simulink model "PPS_Model"  (Simulink 8.2)
settings: Solver=FixedStepDiscrete  SolverMode=SingleTasking  StartTime=0.0  StopTime=inf  FixedStep=1/100  RelTol=1e-3
values from neighbouring files (symbols this model uses):
  dfreq = block.DialogPrm(1).Data    [msfcn_PPS_PlotSpeed.m]    (also in msfcn_PPS_radar_graph.m)
undefined symbols (not defined in the file or in its folder): gray, Rec, SDTV, strel
libraries: simulink x21, visiontextngfix x6, simulink_extras x3, visionsinks x2, visionconversions x2, visionstatistics x1, visionmorphops x1, visionanalysis x1
(part 1 of 2)
settings Model: Creator=Krzysztof  LastModifiedBy=raufk
settings DataIOCC: SaveOutput=off  SaveTime=off
settings OptimizationCC: InlineParams=on  OptimizeBlockIOStorage=off  BufferReuse=off  ExpressionFolding=off  LocalBlockOutputs=off  SimCompilerOptimization=On
settings DebuggingCC: ReadBeforeWriteMsg=DisableAll  WriteAfterWriteMsg=DisableAll  WriteAfterReadMsg=DisableAll  SolverPrmCheckMsg=none  MultiTaskDSMMsg=none  SigSpecEnsureSampleTimeMsg=none  ParameterPrecisionLossMsg=none  FrameProcessingCompatibilityMsg=error  UnknownTsInhSupMsg=none
settings ModelReferenceCC: ModelReferenceNumInstancesAllowed=Single
settings SFSimCC: SimParseCustomCode=off
settings GRTTargetCC: CodeReplacementLibrary=C89/C90 (ANSI)

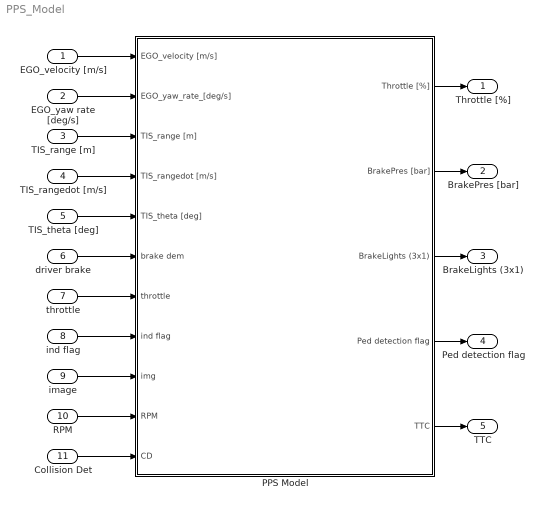
== system PPS_Model ==
  EGO_velocity [m/s] : Inport
  EGO_yaw rate [deg/s] : Inport  Port=2
  TIS_range [m] : Inport  Port=3
  TIS_rangedot [m/s] : Inport  Port=4
  TIS_theta [deg] : Inport  Port=5
  driver brake : Inport  Port=6
  throttle : Inport  Port=7
  ind flag : Inport  Port=8
  image : Inport  Port=9
  RPM : Inport  Port=10
  Collision Det : Inport  Port=11
  PPS Model : Subsystem  mask(PPS Model){MaxSpeed=70, MaxBrakePressure=150, BrakeDelay=100, LaneWidth=3.5, TISMaxRange=40, TISMaxTheta=60, TISfreq=25, TISdet=32, Camfreq=50, Mainfreq=100, DisplaySwitch=on, DisplayFreq=25, RadarSwitch=on, RadarFreq=25}
      mask prompts: MaxSpeed "Vehicle cut-off speed [km/h]"; MaxBrakePressure "Maximum value of braking pressure available [bar]"; BrakeDelay "Braking system delay [ms]"; LaneWidth "Lane width [m]"; TISMaxRange "TIS maximum range [m]"; TISMaxTheta "TIS maximum theta [deg]"; TISfreq "TIS frequency [Hz]"; TISdet "Max. number of Radar detected objects [-]"; Camfreq "Camera frequency [Hz]"; Mainfreq "Compilation sheet frequency [Hz]"; DisplaySwitch "Show EGO parameters visualization"; DisplayFreq "EGO parameters visualization frequency [Hz]"; RadarSwitch "Show radar visualization"; RadarFreq "Radar frequency [Hz]"
      mask help: PreScan Experiment and Pedestrian Protection System parameters
      mask Help: eval('openHelp(8130)')
      mask Callback DisplaySwitch:
      | en = get_param(gcb,'MaskEnables');
      | switch get_param(gcb, 'DisplaySwitch')
      |     case 'off'
      |         en{12} = 'off';
      |     case 'on'
      |         en{12} = 'on';
      | end
      | set_param(gcb,'MaskEnables',en);
      | clear en;
      mask Callback RadarSwitch:
      | en = get_param(gcb,'MaskEnables');
      | switch get_param(gcb, 'RadarSwitch')
      |     case 'off'
      |         en{14} = 'off';
      |     case 'on'
      |         en{14} = 'on';
      | end
      | set_param(gcb,'MaskEnables',en);
      | clear en;
  Throttle [%] : Outport
  BrakePres [bar] : Outport  Port=2
  BrakeLights (3x1) : Outport  Port=3
  Ped detection flag : Outport  Port=4
  TTC : Outport  Port=5
  wires:
  EGO_velocity [m/s]/1 -> PPS Model/1(EGO_velocity [m/s])
  EGO_yaw rate [deg/s]/1 -> PPS Model/2(EGO_yaw_rate_[deg/s])
  TIS_range [m]/1 -> PPS Model/3(TIS_range [m])
  TIS_rangedot [m/s]/1 -> PPS Model/4(TIS_rangedot [m/s])
  TIS_theta [deg]/1 -> PPS Model/5(TIS_theta [deg])
  throttle/1 -> PPS Model/7(throttle)
  ind flag/1 -> PPS Model/8(ind flag)
  image/1 -> PPS Model/9(img)
  PPS Model/1(Throttle [%]) -> Throttle [%]/1
  PPS Model/2(BrakePres [bar]) -> BrakePres [bar]/1
  PPS Model/3(BrakeLights (3x1)) -> BrakeLights (3x1)/1
  PPS Model/5(TTC) -> TTC/1
  driver brake/1 -> PPS Model/6(brake dem)
  RPM/1 -> PPS Model/10(RPM)
  Collision Det/1 -> PPS Model/11(CD)
  PPS Model/4(Ped detection flag) -> Ped detection flag/1

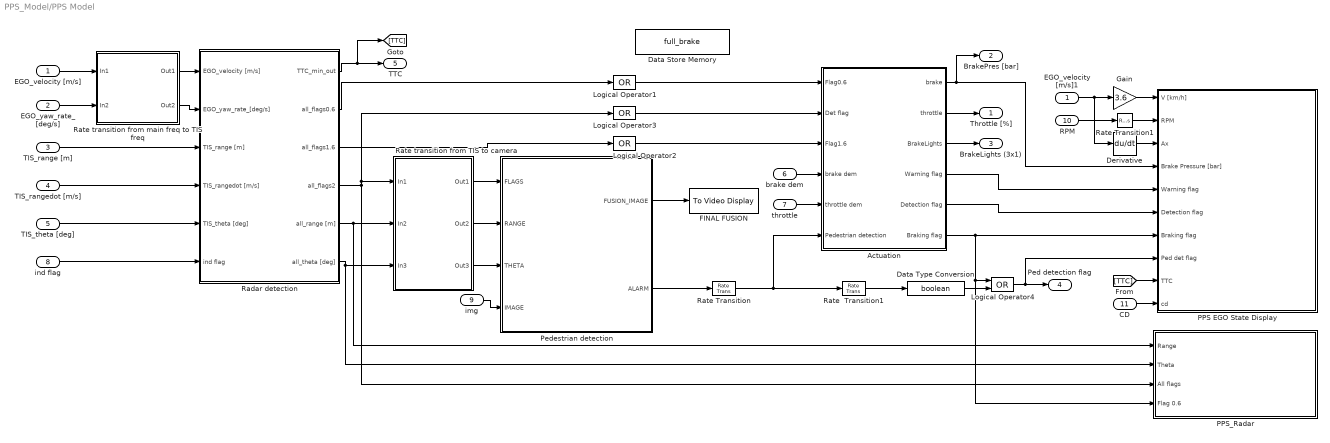
== system PPS_Model/PPS Model ==
  EGO_velocity [m/s] : Inport
  EGO_yaw_rate_[deg/s] : Inport  Port=2  SampleTime=1/Mainfreq
  TIS_range [m] : Inport  Port=3  PortDimensions=TISdet  SampleTime=1/TISfreq
  TIS_rangedot [m/s] : Inport  Port=4  PortDimensions=TISdet  SampleTime=1/TISfreq
  TIS_theta [deg] : Inport  Port=5  PortDimensions=TISdet  SampleTime=1/TISfreq
  brake dem : Inport  Port=6  SampleTime=[0,0]
  throttle : Inport  Port=7  SampleTime=[0,0]
  ind flag : Inport  Port=8  SampleTime=1/TISfreq
  img : Inport  Port=9  PortDimensions=[375 500]  SampleTime=1/Camfreq
  RPM : Inport  Port=10
  CD : Inport  Port=11
  Actuation : Subsystem
  Data Store Memory : DataStoreMemory  DataStoreName=full_brake  ReadBeforeWriteMsg=warning  WriteAfterWriteMsg=warning  WriteAfterReadMsg=warning
  Data Type Conversion : DataTypeConversion  OutDataTypeStr=boolean
  Derivative : Derivative
  EGO_velocity [m/s]1 : InportShadow
  FINAL FUSION : visionsinks/To Video Display  windowSizeMode=True size (1:1)  openAtMdlStart=on  fullScreen=off  videoWindowX=686  videoWindowY=98  saveWindowSize=off  videoWindowWidth=500  videoWindowHeight=375  inputColorFormat=RGB  inputType=Obsolete  imagePorts=One multidimensional signal  OutputDevice=On-screen video monitor  dataOrg=Column-major  isWindowOpen=off
  Gain : Gain  Gain=3.6
  Logical Operator1 : Logic  Operator=OR  Inputs=1  AllPortsSameDT=off  OutDataTypeStr=boolean
  Logical Operator2 : Logic  Operator=OR  Inputs=1  AllPortsSameDT=off  OutDataTypeStr=boolean
  Logical Operator3 : Logic  Operator=OR  Inputs=1  AllPortsSameDT=off  OutDataTypeStr=boolean
  Logical Operator4 : Logic  Operator=OR  AllPortsSameDT=off  OutDataTypeStr=boolean
  PPS EGO State Display : Subsystem  StopFcn=|
      | load('VRU_DisplaySwitch');
      | load('VRU_EGO_State_Coll');
      | load('VRU_EGO_State_BrakeVel');
      | load('VRU_EGO_State_Flag06');
      | s_VRU_DisplaySwitch = VRU_DisplaySwitch(2,end);
      | s_VRU_EGO_State_Coll = VRU_EGO_State_Coll(2,end);
      | s_VRU_EGO_State_BrakeVel = VRU_EGO_State_BrakeVel(2,end);
      | s_VRU_EGO_State_Flag06 = VRU_EGO_State_Flag06(2,end);
      | 
      | if(s_VRU_DisplaySwitch)
      |   CSpanel = findobj('Tag','cs_panel');
      |   CSvalue = findobj('Tag','cs_value');
      |   
      |   if(s_VRU_EGO_State_Coll)
      |      %Collision Occured
      |      set(CSpanel, 'BorderWidth',2, 'ForegroundColor',[0 120/255 0], 'HighlightColor',[0 120/255 0], 'ShadowColor', [0 120/255 0]);
      |      set(CSvalue, 'ForegroundColor',[0 120/255 0], 'String', strcat('Speed reduction', sprintf( ' %.1f ',s_VRU_EGO_State_BrakeVel-s_VRU_EGO_State_Coll), ' km/h'));
      |      set(CSpanel, 'Visible', 'On');
      |      set(CSvalue, 'Visible', 'On');
      |   else
      |     if(s_VRU_EGO_State_Flag06)
      |         % Collision almost occur
      |         set(CSpanel, 'BorderWidth',2, 'ForegroundColor','Green', 'HighlightColor','Green', 'ShadowColor', 'Green');
      |         set(CSvalue, 'ForegroundColor','Green', 'String', 'Collision avoided');
      |         set(CSpanel, 'Visible', 'On');
      |         set(CSvalue, 'Visible', 'On');
      |      else
      |         % No risk of collision
      |         set(CSpanel, 'Visible', 'Off');
      |         set(CSvalue, 'Visible', 'Off');
      |     end
      |   end
      | 
      |   clear CSpanel CSvalue
      | end
      | 
      | PPS_Speed_Profile
      | PPS_TTC_Profile
  PPS_Radar : Subsystem
  Pedestrian detection : Subsystem
  Radar detection : Subsystem
  Rate  Transition1 : RateTransition  Integrity=off  Deterministic=off  OutPortSampleTime=1/min(TISfreq,Camfreq)
  Rate Transition : RateTransition  Integrity=off  Deterministic=off  OutPortSampleTime=[0,0]
  Rate Transition1 : RateTransition  Integrity=off  Deterministic=off  OutPortSampleTime=1/Mainfreq
  Rate transition from TIS to camera : Subsystem
  Rate transition from main freq to TIS freq : Subsystem
  Throttle [%] : Outport
  BrakePres [bar] : Outport  Port=2
  BrakeLights (3x1) : Outport  Port=3
  Ped detection flag : Outport  Port=4  PortDimensions=1
  TTC : Outport  Port=5
  wires:
  TIS_range [m]/1 -> Radar detection/3(TIS_range [m])
  TIS_rangedot [m/s]/1 -> Radar detection/4(TIS_rangedot [m/s])
  TIS_theta [deg]/1 -> Radar detection/5(TIS_theta [deg])
  ind flag/1 -> Radar detection/6(ind flag)
  EGO_velocity [m/s]/1 -> Rate transition from main freq to TIS freq/1(In1)
  EGO_yaw_rate_[deg/s]/1 -> Rate transition from main freq to TIS freq/2(In2)
  Rate transition from main freq to TIS freq/1(Out1) -> Radar detection/1(EGO_velocity [m/s])
  Rate transition from main freq to TIS freq/2(Out2) -> Radar detection/2(EGO_yaw_rate_[deg/s])
  throttle/1 -> Actuation/5(throttle dem)
  brake dem/1 -> Actuation/4(brake dem)
  Radar detection/1(TTC_min_out) -> TTC/1, [TTC]
  Radar detection/2(all_flags0.6) -> Logical Operator1/1
  Rate Transition/1 -> Actuation/6(Pedestrian detection), Rate  Transition1/1
  Rate  Transition1/1 -> Data Type Conversion/1
  Radar detection/4(all_flags2) -> Rate transition from TIS to camera/1(In1), Logical Operator3/1, PPS_Radar/3(All flags)
  Radar detection/5(all_range [m]) -> Rate transition from TIS to camera/2(In2), PPS_Radar/1(Range)
  Radar detection/6(all_theta [deg]) -> PPS_Radar/2(Theta), Rate transition from TIS to camera/3(In3)
  Radar detection/3(all_flags1.6) -> Logical Operator2/1
  Actuation/1(brake) -> BrakePres [bar]/1, PPS EGO State Display/4(Brake Pressure [bar])
  Actuation/2(throttle) -> Throttle [%]/1
  Actuation/3(BrakeLights) -> BrakeLights (3x1)/1
  Actuation/6(Braking flag) -> PPS EGO State Display/7(Braking flag), Logical Operator4/1, PPS_Radar/4(Flag 0.6)
  img/1 -> Pedestrian detection/4(IMAGE)
  Pedestrian detection/1(FUSION_IMAGE) -> FINAL FUSION/1
  Rate transition from TIS to camera/1(Out1) -> Pedestrian detection/1(FLAGS)
  Rate transition from TIS to camera/2(Out2) -> Pedestrian detection/2(RANGE)
  Rate transition from TIS to camera/3(Out3) -> Pedestrian detection/3(THETA)
  Logical Operator1/1 -> Actuation/1(Flag0.6)
  Logical Operator2/1 -> Actuation/3(Flag1.6)
  Data Type Conversion/1 -> Logical Operator4/2
  Logical Operator4/1 -> PPS EGO State Display/8(Ped det flag), Ped detection flag/1
  Logical Operator3/1 -> Actuation/2(Det flag)
  EGO_velocity [m/s]1/1 -> Gain/1, Derivative/1
  Gain/1 -> PPS EGO State Display/1(V [km/h])
  RPM/1 -> Rate Transition1/1
  Derivative/1 -> PPS EGO State Display/3(Ax)
  CD/1 -> PPS EGO State Display/10(cd)
  [TTC] -> PPS EGO State Display/9(TTC)
  Actuation/4(Warning flag) -> PPS EGO State Display/5(Warning flag)
  Actuation/5(Detection flag) -> PPS EGO State Display/6(Detection flag)
  Rate Transition1/1 -> PPS EGO State Display/2(RPM)
  Pedestrian detection/2(ALARM) -> Rate Transition/1

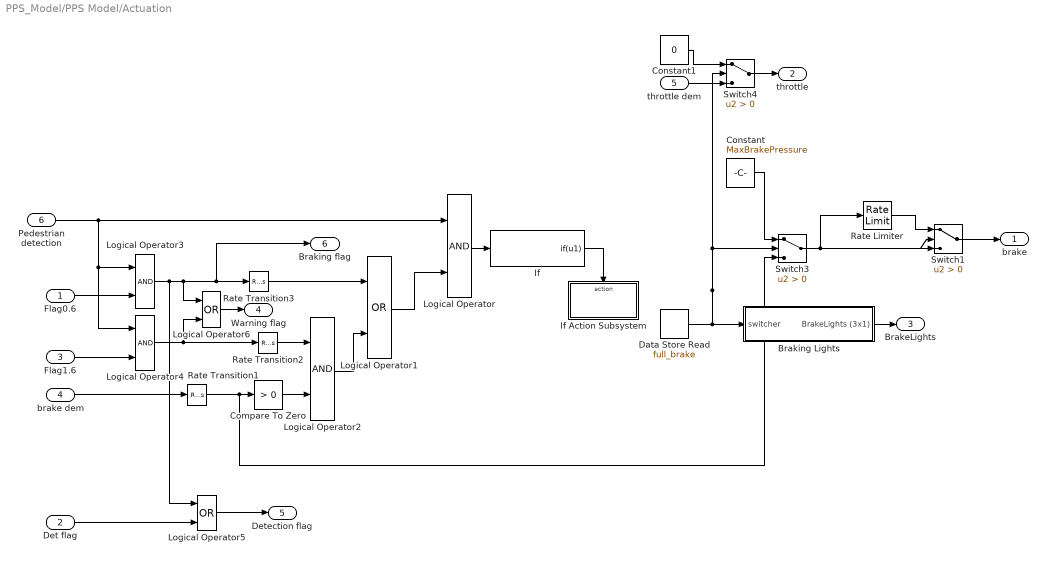
== system PPS_Model/PPS Model/Actuation ==
  Flag0.6 : Inport
  Det flag : Inport  Port=2
  Flag1.6 : Inport  Port=3
  brake dem : Inport  Port=4
  throttle dem : Inport  Port=5
  Pedestrian detection : Inport  Port=6
  Braking Lights : Subsystem
  Compare To Zero : simulink/Logic and Bit Operations/Compare To Zero  relop=>  OutDataTypeStr=uint8
  Constant : Constant  Value=MaxBrakePressure  SampleTime=[0,0]
  Constant1 : Constant  Value=0  SampleTime=[0,0]
  Data Store Read : DataStoreRead  DataStoreName=full_brake  SampleTime=1/Mainfreq
  If : If  IfExpression=u1  ShowElse=off
  If Action Subsystem : Subsystem  TreatAsAtomicUnit=on
  Logical Operator : Logic  AllPortsSameDT=off  OutDataTypeStr=boolean  SampleTime=[0,0]
  Logical Operator1 : Logic  Operator=OR  AllPortsSameDT=off  OutDataTypeStr=boolean  SampleTime=[0,0]
  Logical Operator2 : Logic  AllPortsSameDT=off  OutDataTypeStr=boolean  SampleTime=[0,0]
  Logical Operator3 : Logic  AllPortsSameDT=off  OutDataTypeStr=boolean  SampleTime=1/TISfreq
  Logical Operator4 : Logic  AllPortsSameDT=off  OutDataTypeStr=boolean  SampleTime=1/TISfreq
  Logical Operator5 : Logic  Operator=OR  AllPortsSameDT=off  OutDataTypeStr=boolean  SampleTime=1/TISfreq
  Logical Operator6 : Logic  Operator=OR  AllPortsSameDT=off  OutDataTypeStr=boolean  SampleTime=1/TISfreq
  Rate Limiter : RateLimiter  RisingSlewLimit=1000*0.9*MaxBrakePressure/BrakeDelay  FallingSlewLimit=-inf  SampleTimeMode=inherited
  Rate Transition1 : RateTransition  Integrity=off  OutPortSampleTime=[0,0]
  Rate Transition2 : RateTransition  Integrity=off  OutPortSampleTime=[0,0]
  Rate Transition3 : RateTransition  Integrity=off  OutPortSampleTime=[0,0]
  Switch1 : Switch  Criteria=u2 > Threshold  SampleTime=[0,0]
  Switch3 : Switch  Criteria=u2 > Threshold  SampleTime=[0,0]
  Switch4 : Switch  Criteria=u2 > Threshold  SampleTime=[0,0]
  brake : Outport  SampleTime=[0,0]
  throttle : Outport  Port=2  SampleTime=[0,0]
  BrakeLights : Outport  Port=3  SampleTime=1/Mainfreq
  Warning flag : Outport  Port=4
  Detection flag : Outport  Port=5
  Braking flag : Outport  Port=6
  wires:
  Pedestrian detection/1 -> Logical Operator3/1, Logical Operator4/1, Logical Operator/1
  Logical Operator1/1 -> Logical Operator/2
  Logical Operator2/1 -> Logical Operator1/2
  Compare To Zero/1 -> Logical Operator2/2
  Constant/1 -> Switch3/1
  Constant1/1 -> Switch4/1
  Switch4/1 -> throttle/1
  throttle dem/1 -> Switch4/3
  Braking Lights/1(BrakeLights (3x1)) -> BrakeLights/1
  brake dem/1 -> Rate Transition1/1
  Rate Transition1/1 -> Compare To Zero/1, Switch3/3
  Rate Transition2/1 -> Logical Operator2/1
  Rate Transition3/1 -> Logical Operator1/1
  Switch3/1 -> Switch1/3, Rate Limiter/1
  Rate Limiter/1 -> Switch1/1
  Switch1/1 -> brake/1
  Logical Operator3/1 -> Rate Transition3/1, Braking flag/1, Logical Operator6/1, Logical Operator5/1
  Logical Operator4/1 -> Rate Transition2/1, Logical Operator6/2
  Flag0.6/1 -> Logical Operator3/2
  Flag1.6/1 -> Logical Operator4/2
  Logical Operator6/1 -> Warning flag/1
  Det flag/1 -> Logical Operator5/2
  Logical Operator5/1 -> Detection flag/1
  Logical Operator/1 -> If/1
  Data Store Read/1 -> Braking Lights/1(switcher), Switch3/2, Switch1/2, Switch4/2
  If/1 -> If Action Subsystem/Action

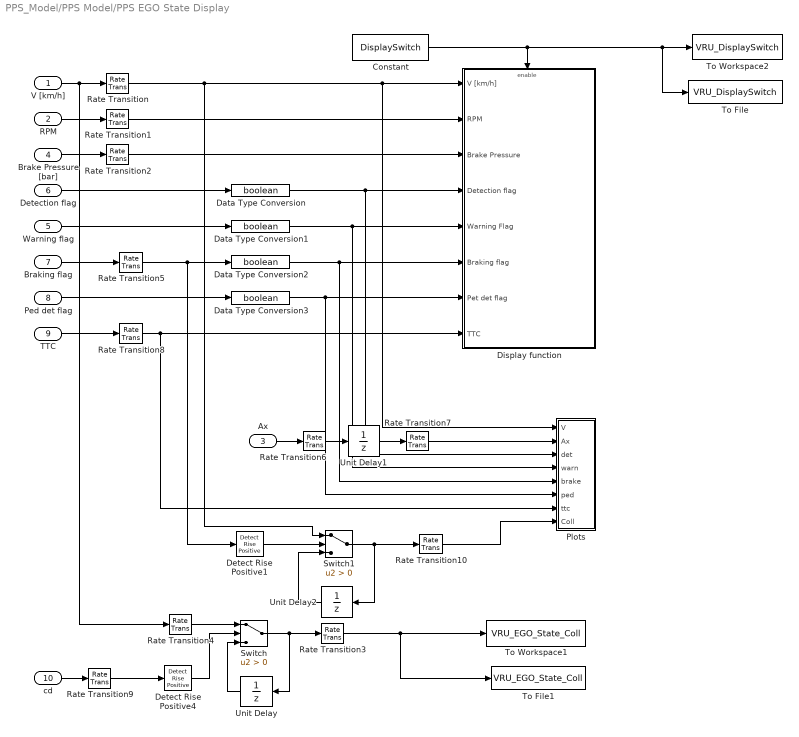
== system PPS_Model/PPS Model/PPS EGO State Display ==
  V [km/h] : Inport
  RPM : Inport  Port=2
  Ax : Inport  Port=3  SampleTime=[0,0]
  Brake Pressure [bar] : Inport  Port=4
  Warning flag : Inport  Port=5  OutDataTypeStr=boolean
  Detection flag : Inport  Port=6  OutDataTypeStr=boolean
  Braking flag : Inport  Port=7  OutDataTypeStr=boolean
  Ped det flag : Inport  Port=8  OutDataTypeStr=boolean
  TTC : Inport  Port=9
  cd : Inport  Port=10  OutDataTypeStr=boolean
  Constant : Constant  Value=DisplaySwitch
  Data Type Conversion{,1..3} (4 alike) : DataTypeConversion  OutDataTypeStr=boolean
  Detect Rise Positive1 : simulink/Logic and Bit Operations/Detect Rise Positive  vinit=0  InputProcessing=Inherited  OutDataTypeStr=uint8
  Detect Rise Positive4 : simulink/Logic and Bit Operations/Detect Rise Positive  vinit=0  InputProcessing=Inherited  OutDataTypeStr=uint8
  Display function : Subsystem
  Plots : Subsystem
      mask help:
      | The block calls functions:
      | * PPS_Speed_Profile
      | * PPS_TTC_Profile
      | to generate plots at the end of the simulation.
      | See stop callback of the block for more details.
  Rate Transition{,1..2,5,7..8} (6 alike) : RateTransition  Integrity=off  OutPortSampleTime=1/DisplayFreq
  Rate Transition10 : RateTransition  Integrity=off  OutPortSampleTime=[0,0]
  Rate Transition3 : RateTransition  Integrity=off  OutPortSampleTime=[0,0]
  Rate Transition4 : RateTransition  Integrity=off  OutPortSampleTime=1/Mainfreq
  Rate Transition6 : RateTransition  Integrity=off  OutPortSampleTimeOpt=Inherit  OutPortSampleTime=1/dfreq
  Rate Transition9 : RateTransition  Integrity=off  OutPortSampleTime=1/Mainfreq
  Switch : Switch  Criteria=u2 > Threshold  SampleTime=1/Mainfreq
  Switch1 : Switch  Criteria=u2 > Threshold  SampleTime=1/Mainfreq
  To File : ToFile  Filename=VRU_DisplaySwitch  MatrixName=VRU_DisplaySwitch  SampleTime=1/Mainfreq
  To File1 : ToFile  Filename=VRU_EGO_State_Coll  MatrixName=VRU_EGO_State_Coll  SampleTime=1/Mainfreq
  To Workspace1 : ToWorkspace  VariableName=VRU_EGO_State_Coll  SampleTime=1/Mainfreq
      settings: MaxDataPoints=1
  To Workspace2 : ToWorkspace  VariableName=VRU_DisplaySwitch  SampleTime=1/Mainfreq
      settings: MaxDataPoints=1
  Unit Delay : UnitDelay  SampleTime=1/Mainfreq
  Unit Delay1 : UnitDelay  SampleTime=-1
  Unit Delay2 : UnitDelay  SampleTime=1/Mainfreq
  wires:
  RPM/1 -> Rate Transition1/1
  Brake Pressure [bar]/1 -> Rate Transition2/1
  V [km/h]/1 -> Rate Transition/1, Rate Transition4/1
  Warning flag/1 -> Data Type Conversion1/1
  Ped det flag/1 -> Data Type Conversion3/1
  TTC/1 -> Rate Transition8/1
  Detection flag/1 -> Data Type Conversion/1
  Rate Transition/1 -> Display function/1(V [km/h]), Plots/1(V), Switch1/1
  Rate Transition1/1 -> Display function/2(RPM)
  Rate Transition3/1 -> To File1/1, To Workspace1/1
  cd/1 -> Rate Transition9/1
  Switch/1 -> Unit Delay/1, Rate Transition3/1
  Unit Delay/1 -> Switch/3
  Rate Transition4/1 -> Switch/1
  Detect Rise Positive4/1 -> Switch/2
  Braking flag/1 -> Rate Transition5/1
  Rate Transition5/1 -> Data Type Conversion2/1, Detect Rise Positive1/1
  Ax/1 -> Rate Transition6/1
  Unit Delay1/1 -> Rate Transition7/1
  Rate Transition6/1 -> Unit Delay1/1
  Rate Transition2/1 -> Display function/3(Brake Pressure)
  Rate Transition7/1 -> Plots/2(Ax)
  Rate Transition8/1 -> Plots/7(ttc), Display function/8(TTC)
  Rate Transition9/1 -> Detect Rise Positive4/1
  Data Type Conversion3/1 -> Plots/6(ped), Display function/7(Pet det flag)
  Data Type Conversion2/1 -> Display function/6(Braking flag), Plots/5(brake)
  Data Type Conversion1/1 -> Plots/4(warn), Display function/5(Warning Flag)
  Data Type Conversion/1 -> Plots/3(det), Display function/4(Detection flag)
  Constant/1 -> Display function/Enable, To File/1, To Workspace2/1
  Detect Rise Positive1/1 -> Switch1/2
  Switch1/1 -> Unit Delay2/1, Rate Transition10/1
  Unit Delay2/1 -> Switch1/3
  Rate Transition10/1 -> Plots/8(Coll)

== system PPS_Model/PPS Model/PPS_Radar ==
  Range : Inport
  Theta : Inport  Port=2
  All flags : Inport  Port=3  OutDataTypeStr=boolean
  Flag 0.6 : Inport  Port=4  OutDataTypeStr=boolean
  Constant : Constant  Value=RadarSwitch
  Radar : Subsystem
  Rate Transition{1..4} (4 alike) : RateTransition  Integrity=off  Deterministic=off  OutPortSampleTime=1/RadarFreq
  wires:
  Range/1 -> Rate Transition1/1
  Theta/1 -> Rate Transition2/1
  All flags/1 -> Rate Transition3/1
  Flag 0.6/1 -> Rate Transition4/1
  Rate Transition1/1 -> Radar/1(Range)
  Rate Transition2/1 -> Radar/2(Theta)
  Rate Transition3/1 -> Radar/3(All flags)
  Rate Transition4/1 -> Radar/4(Flag 0.6)
  Constant/1 -> Radar/Enable

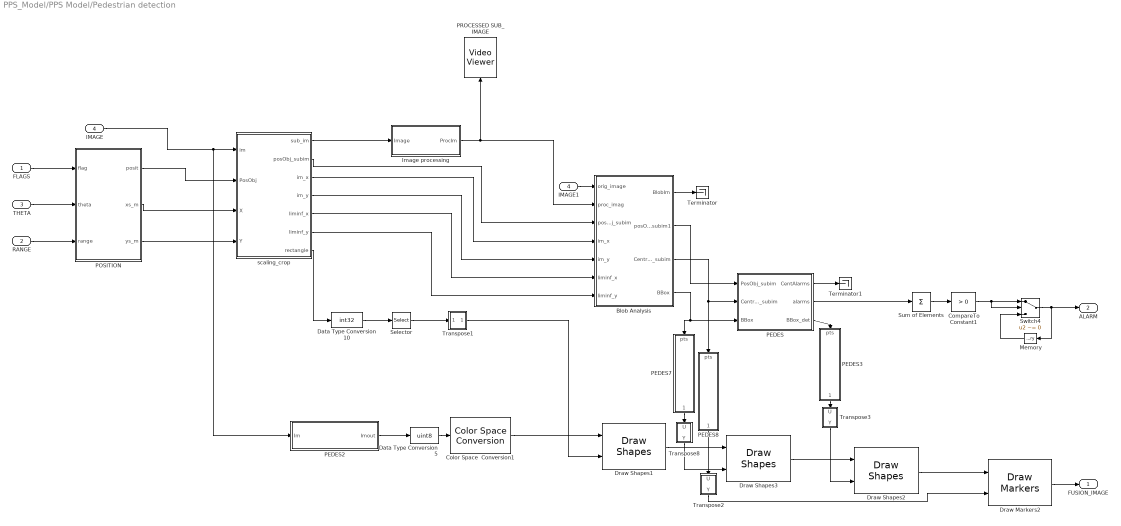
== system PPS_Model/PPS Model/Pedestrian detection ==
  FLAGS : Inport  OutDataTypeStr=boolean
  RANGE : Inport  Port=2  PortDimensions=TISdet
  THETA : Inport  Port=3
  IMAGE : Inport  Port=4  OutDataTypeStr=uint8  PortDimensions=[375 500]
  Blob Analysis : Subsystem
  Color Space  Conversion1 : visionconversions/Color Space  Conversion  conversion=Obsolete  conversionActive=Y'CbCr to R'G'B'  wp_str=D65  rec=Rec. 601 (SDTV)  sys=1125/60/2:1  imagePorts=One multidimensional signal
  CompareTo Constant1 : simulink/Logic and Bit Operations/Compare To Constant  relop=>  const=0  OutDataTypeStr=uint8
  Data Type Conversion10 : DataTypeConversion  OutDataTypeStr=int32
  Data Type Conversion5 : DataTypeConversion  OutDataTypeStr=uint8
  Draw Markers2 : visiontextngfix/Draw Markers  shape=X-mark  size=3  fill=on  fillClrSource=Specify via dialog  display=White  intensity=200  color=[200 255 100]  opacity=0.9  viewport=Entire image  antialiasing=on  inType=Obsolete  imagePorts=One multidimensional signal  prodOutputMode=Binary point scaling  prodOutputWordLength=32  prodOutputFracLength=14  memoryMode=Specify word length  memoryWordLength=16  memoryFracLength=14  roundingMode=Floor  overflowMode=off
  Draw Shapes1 : visiontextngfix/Draw Shapes  shape=Rectangles  fill=off  fillClrSource=Specify via dialog  display=White  intensity=200  color=[255 0 0]  opacity=0.5  viewport=Entire image  antialiasing=off  inType=Obsolete  imagePorts=One multidimensional signal  prodOutputMode=Binary point scaling  prodOutputWordLength=32  prodOutputFracLength=14  memoryMode=Specify word length  memoryWordLength=16  memoryFracLength=14  roundingMode=Floor  overflowMode=off
  Draw Shapes2 : visiontextngfix/Draw Shapes  shape=Rectangles  fill=on  fillClrSource=Specify via dialog  display=White  intensity=200  color=[255 0 0]  opacity=0.5  viewport=Entire image  antialiasing=off  inType=Obsolete  imagePorts=One multidimensional signal  prodOutputMode=Binary point scaling  prodOutputWordLength=32  prodOutputFracLength=14  memoryMode=Specify word length  memoryWordLength=16  memoryFracLength=14  roundingMode=Floor  overflowMode=off
  Draw Shapes3 : visiontextngfix/Draw Shapes  shape=Rectangles  fill=off  fillClrSource=Specify via dialog  display=User-specified value  intensity=200  color=[255 0 0]  opacity=0.5  viewport=Entire image  antialiasing=off  inType=Obsolete  imagePorts=One multidimensional signal  prodOutputMode=Binary point scaling  prodOutputWordLength=32  prodOutputFracLength=14  memoryMode=Specify word length  memoryWordLength=16  memoryFracLength=14  roundingMode=Floor  overflowMode=off
  IMAGE1 : InportShadow  Port=4  OutDataTypeStr=uint8  PortDimensions=[375 500]
  Image processing : Subsystem
  Memory : Memory
  PEDES : MATLAB Function  TreatAsAtomicUnit=on
      settings: PermitHierarchicalResolution=ParametersOnly
  PEDES2 : MATLAB Function  TreatAsAtomicUnit=on
      settings: PermitHierarchicalResolution=ParametersOnly
  PEDES3 : MATLAB Function  TreatAsAtomicUnit=on
      settings: PermitHierarchicalResolution=ParametersOnly
  PEDES7 : MATLAB Function  TreatAsAtomicUnit=on
      settings: PermitHierarchicalResolution=ParametersOnly
  PEDES8 : MATLAB Function  TreatAsAtomicUnit=on
      settings: PermitHierarchicalResolution=ParametersOnly
  POSITION : MATLAB Function  TreatAsAtomicUnit=on
      settings: PermitHierarchicalResolution=ParametersOnly
  PROCESSED SUB_IMAGE : visionsinks/Video Viewer  inputType=Obsolete7b  imagePorts=One multidimensional signal  useColorMap=off  colormapValue=gray(256)  specRange=off  minInputVal=0  maxInputVal=255  FigPos=[546 1020 501 324]  AxisZoom=on  trueSizedOnce=off  OpenAtMdlStart=on  DefaultConfigurationName=vipscopes.VideoViewerScopeCfg
  Selector : Selector  InputPortWidth=4  IndexOptions=Index vector (dialog)  Indices=[2, 1, 4, 3]  OutputSizes=1
  Sum of Elements : Sum  Inputs=+
  Switch4 : Switch  Criteria=u2 ~= 0
  Terminator : Terminator
  Terminator1 : Terminator
  Transpose1 : Subsystem
  Transpose2 : Subsystem
  Transpose3 : Subsystem
  Transpose8 : Subsystem
  scaling_crop : MATLAB Function  TreatAsAtomicUnit=on
      settings: PermitHierarchicalResolution=ParametersOnly
  FUSION_IMAGE : Outport
  ALARM : Outport  Port=2
  wires:
  THETA/1 -> POSITION/2(theta)
  FLAGS/1 -> POSITION/1(flag)
  RANGE/1 -> POSITION/3(range)
  Blob Analysis/3(Centroid_subim) -> PEDES/2(Centroid_subim), PEDES8/1(pts)
  PEDES/2(alarms) -> Sum of Elements/1
  Blob Analysis/4(BBox) -> PEDES/3(BBox), PEDES7/1(pts)
  Switch4/1 -> ALARM/1, Memory/1
  Memory/1 -> Switch4/3
  Sum of Elements/1 -> CompareTo Constant1/1
  CompareTo Constant1/1 -> Switch4/1, Switch4/2
  Blob Analysis/2(posObj_subim1) -> PEDES/1(PosObj_subim)
  scaling_crop/6(liminf_y) -> Blob Analysis/7(liminf_y)
  scaling_crop/7(rectangle) -> Data Type Conversion10/1
  PEDES2/1(Imout) -> Data Type Conversion5/1
  Data Type Conversion5/1 -> Color Space  Conversion1/1
  Color Space  Conversion1/1 -> Draw Shapes1/1
  Draw Shapes1/1 -> Draw Shapes3/1
  Draw Shapes3/1 -> Draw Shapes2/1
  Draw Shapes2/1 -> Draw Markers2/1
  POSITION/2(xs_m) -> scaling_crop/3(X)
  POSITION/3(ys_m) -> scaling_crop/4(Y)
  POSITION/1(posit) -> scaling_crop/2(PosObj)
  IMAGE/1 -> scaling_crop/1(im), PEDES2/1(Im)
  scaling_crop/1(sub_im) -> Image processing/1(Image)
  scaling_crop/2(posObj_subim) -> Blob Analysis/3(posObj_subim)
  scaling_crop/3(im_x) -> Blob Analysis/4(im_x)
  scaling_crop/4(im_y) -> Blob Analysis/5(im_y)
  scaling_crop/5(liminf_x) -> Blob Analysis/6(liminf_x)
  PEDES/3(BBox_det) -> PEDES3/1(pts)
  Draw Markers2/1 -> FUSION_IMAGE/1
  Image processing/1(ProcIm) -> Blob Analysis/2(proc_imag), PROCESSED SUB_IMAGE/1
  Transpose1/1(Y) -> Draw Shapes1/2
  Selector/1 -> Transpose1/1(U)
  Data Type Conversion10/1 -> Selector/1
  Transpose3/1(Y) -> Draw Shapes2/2
  Transpose2/1(Y) -> Draw Markers2/2
  Transpose8/1(Y) -> Draw Shapes3/2
  PEDES7/1(inpoints) -> Transpose8/1(U)
  PEDES8/1(inpoints) -> Transpose2/1(U)
  PEDES3/1(inpoints) -> Transpose3/1(U)
  Blob Analysis/1(BlobIm) -> Terminator/1
  PEDES/1(CentAlarms) -> Terminator1/1
  IMAGE1/1 -> Blob Analysis/1(orig_image)

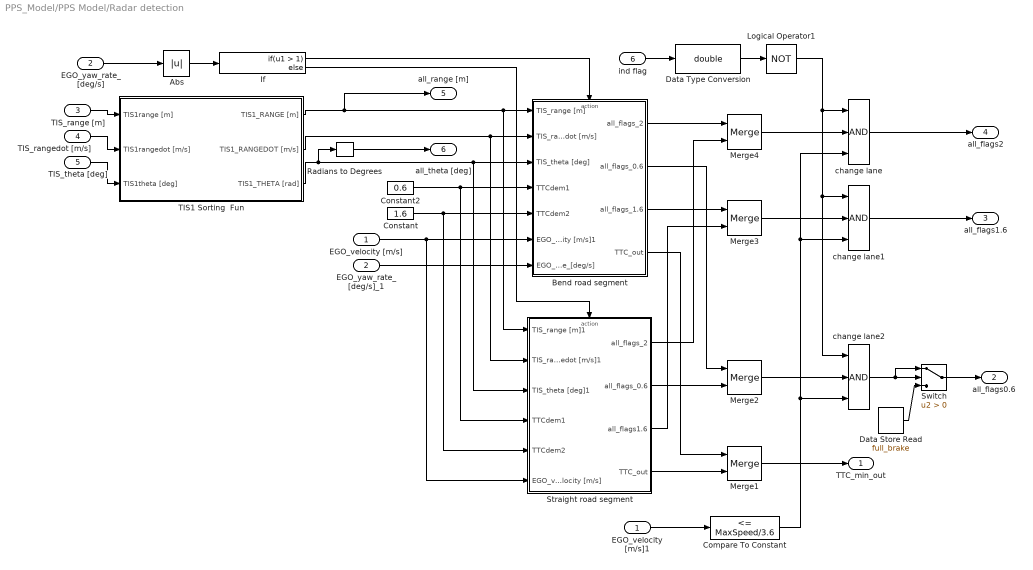
== system PPS_Model/PPS Model/Radar detection ==
  EGO_velocity [m/s] : Inport
  EGO_yaw_rate_[deg/s] : Inport  Port=2
  TIS_range [m] : Inport  Port=3  PortDimensions=TISdet
  TIS_rangedot [m/s] : Inport  Port=4  PortDimensions=TISdet
  TIS_theta [deg] : Inport  Port=5  PortDimensions=TISdet
  ind flag : Inport  Port=6
  Abs : Abs
  Bend road segment : Subsystem  TreatAsAtomicUnit=on
  Compare To Constant : simulink/Logic and Bit Operations/Compare To Constant  relop=<=  const=MaxSpeed/3.6  OutDataTypeStr=uint8
  Constant : Constant  Value=1.6
  Constant2 : Constant  Value=0.6
  Data Store Read : DataStoreRead  DataStoreName=full_brake  SampleTime=1/Mainfreq
  Data Type Conversion : DataTypeConversion  OutDataTypeStr=double
  EGO_velocity [m/s]1 : InportShadow
  EGO_yaw_rate_[deg/s]_1 : InportShadow  Port=2
  If : If  IfExpression=u1 > 1  SampleTime=1/TISfreq
  Logical Operator1 : Logic  Operator=NOT  AllPortsSameDT=off  OutDataTypeStr=boolean
  Merge{1..4} (4 alike) : Merge
  Radians to Degrees : simulink_extras/Transformations/Radians to Degrees
  Straight road segment : Subsystem  TreatAsAtomicUnit=on
  Switch : Switch  Criteria=u2 > Threshold
  TIS1 Sorting  Fun : Subsystem
  change lane : Logic  Inputs=3  AllPortsSameDT=off  OutDataTypeStr=boolean
  change lane1 : Logic  Inputs=3  AllPortsSameDT=off  OutDataTypeStr=boolean
  change lane2 : Logic  Inputs=3  AllPortsSameDT=off  OutDataTypeStr=boolean
  TTC_min_out : Outport
  all_flags0.6 : Outport  Port=2
  all_flags1.6 : Outport  Port=3
  all_flags2 : Outport  Port=4
  all_range [m] : Outport  Port=5
  all_theta [deg] : Outport  Port=6
  wires:
  TIS_range [m]/1 -> TIS1 Sorting  Fun/1(TIS1range [m])
  TIS_rangedot [m/s]/1 -> TIS1 Sorting  Fun/2(TIS1rangedot [m/s])
  TIS_theta [deg]/1 -> TIS1 Sorting  Fun/3(TIS1theta [deg])
  EGO_yaw_rate_[deg/s]/1 -> Abs/1
  If/1 -> Bend road segment/Action
  Abs/1 -> If/1
  TIS1 Sorting  Fun/1(TIS1_RANGE [m]) -> Bend road segment/1(TIS_range [m]), Straight road segment/1(TIS_range [m]1), all_range [m]/1
  TIS1 Sorting  Fun/2(TIS1_RANGEDOT [m/s]) -> Bend road segment/2(TIS_rangedot [m/s]), Straight road segment/2(TIS_rangedot [m/s]1)
  TIS1 Sorting  Fun/3(TIS1_THETA [rad]) -> Bend road segment/3(TIS_theta [deg]), Straight road segment/3(TIS_theta [deg]1), Radians to Degrees/1
  If/2 -> Straight road segment/Action
  Constant2/1 -> Bend road segment/4(TTCdem1), Straight road segment/4(TTCdem1)
  Constant/1 -> Bend road segment/5(TTCdem2), Straight road segment/5(TTCdem2)
  EGO_velocity [m/s]/1 -> Bend road segment/6(EGO_velocity [m/s]1), Straight road segment/6(EGO_velocity [m/s])
  EGO_yaw_rate_[deg/s]_1/1 -> Bend road segment/7(EGO_yaw_rate_[deg/s])
  ind flag/1 -> Data Type Conversion/1
  Bend road segment/2(all_flags_0.6) -> Merge2/1
  Straight road segment/2(all_flags_0.6) -> Merge2/2
  Straight road segment/3(all_flags1.6) -> Merge3/2
  Bend road segment/3(all_flags_1.6) -> Merge3/1
  Radians to Degrees/1 -> all_theta [deg]/1
  Data Type Conversion/1 -> Logical Operator1/1
  Straight road segment/4(TTC_out) -> Merge1/2
  Bend road segment/4(TTC_out) -> Merge1/1
  Merge1/1 -> TTC_min_out/1
  Bend road segment/1(all_flags_2) -> Merge4/1
  Straight road segment/1(all_flags_2) -> Merge4/2
  Merge4/1 -> change lane/2
  Logical Operator1/1 -> change lane/1, change lane2/1, change lane1/1
  Merge3/1 -> change lane1/2
  Merge2/1 -> change lane2/2
  change lane/1 -> all_flags2/1
  change lane2/1 -> Switch/2, Switch/1
  Switch/1 -> all_flags0.6/1
  EGO_velocity [m/s]1/1 -> Compare To Constant/1
  Compare To Constant/1 -> change lane2/3, change lane1/3, change lane/3
  change lane1/1 -> all_flags1.6/1
  Data Store Read/1 -> Switch/3

== system PPS_Model/PPS Model/Rate transition from TIS to camera ==
  In1 : Inport
  In2 : Inport  Port=2
  In3 : Inport  Port=3
  Rate Transition1 : RateTransition  Integrity=off  Deterministic=off  X0=zeros(TISdet,1)  OutPortSampleTime=1/Camfreq
  Rate Transition2 : RateTransition  Integrity=off  Deterministic=off  X0=zeros(TISdet,1)  OutPortSampleTime=1/Camfreq
  Rate Transition3 : RateTransition  Integrity=off  Deterministic=off  X0=zeros(TISdet,1)  OutPortSampleTime=1/Camfreq
  Out1 : Outport
  Out2 : Outport  Port=2
  Out3 : Outport  Port=3
  wires:
  In1/1 -> Rate Transition3/1
  In2/1 -> Rate Transition1/1
  In3/1 -> Rate Transition2/1
  Rate Transition3/1 -> Out1/1
  Rate Transition1/1 -> Out2/1
  Rate Transition2/1 -> Out3/1

== system PPS_Model/PPS Model/Rate transition from main freq to TIS freq ==
  In1 : Inport
  In2 : Inport  Port=2
  Rate Transition1 : RateTransition  Integrity=off  Deterministic=off  OutPortSampleTime=1/TISfreq
  Rate Transition2 : RateTransition  Integrity=off  Deterministic=off  OutPortSampleTime=1/TISfreq
  Out1 : Outport
  Out2 : Outport  Port=2
  wires:
  Rate Transition1/1 -> Out2/1
  In2/1 -> Rate Transition1/1
  In1/1 -> Rate Transition2/1
  Rate Transition2/1 -> Out1/1

== system PPS_Model/PPS Model/Actuation/Braking Lights ==
  note: === Braking lights block ===
      |
      |    - according to brake pressure, lights up braking lights of the actor,
      |    - the signal is a 3x1 vector:
      |      = first        value - left braking light,
      |      = second value - middle braking light,
      |      = third       value - right braking light.
  switcher : Inport
  Add : Sum
  Constant : Constant
  Constant1 : Constant  Value=0
  Mux : Mux  Inputs=3
  Pulse Generator : DiscretePulseGenerator  PulseType=Time based  Period=0.6  PulseWidth=50  PhaseDelay=0.3
  Rate Transition3 : RateTransition  Integrity=off  Deterministic=off  OutPortSampleTime=[0,0]
  Switch : Switch  Criteria=u2 > Threshold
  Switch1 : Switch  Criteria=u2 > Threshold
  Switch2 : Switch  Criteria=u2 > Threshold
  Unary Minus : UnaryMinus
  BrakeLights (3x1) : Outport
  wires:
  Mux/1 -> BrakeLights (3x1)/1
  switcher/1 -> Switch/2, Switch1/2, Switch2/2
  Constant/1 -> Switch/1, Add/2
  Switch/1 -> Switch1/3, Switch2/3, Mux/2
  Constant1/1 -> Switch/3
  Switch2/1 -> Mux/1
  Switch1/1 -> Mux/3
  Pulse Generator/1 -> Rate Transition3/1
  Add/1 -> Switch1/1
  Unary Minus/1 -> Add/1
  Rate Transition3/1 -> Unary Minus/1, Switch2/1

== system PPS_Model/PPS Model/Actuation/If Action Subsystem ==
  Action Port : ActionPort  ActionType=then
  Constant1 : Constant  SampleTime=[0,0]
  Data Store Write : DataStoreWrite  DataStoreName=full_brake
  wires:
  Constant1/1 -> Data Store Write/1

== system PPS_Model/PPS Model/PPS EGO State Display/Display function ==
  V [km/h] : Inport
  RPM : Inport  Port=2
  Brake Pressure : Inport  Port=3
  Detection flag : Inport  Port=4
  Warning Flag : Inport  Port=5
  Braking flag : Inport  Port=6
  Pet det flag : Inport  Port=7
  TTC : Inport  Port=8
  Enable : EnablePort
  Brake Pressure [bar]2 : Gain  Gain=100/MaxBrakePressure
  EGO Vehicle state display : M-S-Function  FunctionName=msfcn_PPS_PlotSpeed  Parameters=DisplayFreq DisplaySwitch
  Rounding Function2 : Rounding  Operator=round
  Rounding Function3 : Rounding  Operator=round
  wires:
  Brake Pressure [bar]2/1 -> Rounding Function3/1
  Rounding Function3/1 -> EGO Vehicle state display/3
  Rounding Function2/1 -> EGO Vehicle state display/2
  V [km/h]/1 -> EGO Vehicle state display/1
  Detection flag/1 -> EGO Vehicle state display/4
  Warning Flag/1 -> EGO Vehicle state display/5
  Braking flag/1 -> EGO Vehicle state display/6
  Pet det flag/1 -> EGO Vehicle state display/7
  TTC/1 -> EGO Vehicle state display/8
  RPM/1 -> Rounding Function2/1
  Brake Pressure/1 -> Brake Pressure [bar]2/1

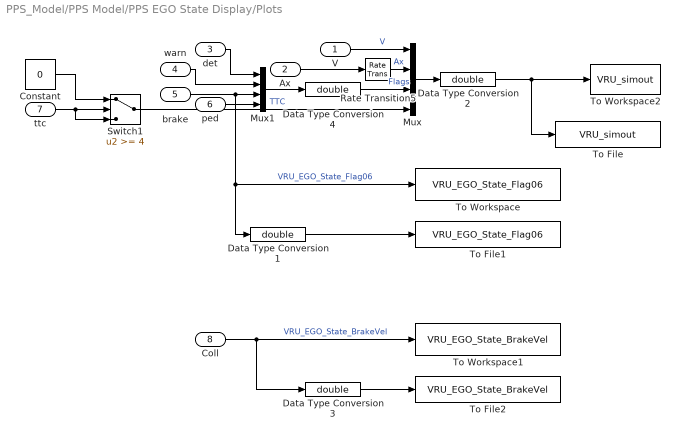
== system PPS_Model/PPS Model/PPS EGO State Display/Plots ==
  V : Inport
  Ax : Inport  Port=2  SampleTime=[0,0]
  det : Inport  Port=3
  warn : Inport  Port=4
  brake : Inport  Port=5
  ped : Inport  Port=6
  ttc : Inport  Port=7
  Coll : Inport  Port=8
  Constant : Constant  Value=0
  Data Type Conversion{1..4} (4 alike) : DataTypeConversion  OutDataTypeStr=double
  Mux : Mux
  Mux1 : Mux
  Rate Transition5 : RateTransition  Integrity=off  OutPortSampleTime=1/DisplayFreq
  Switch1 : Switch  Threshold=4
  To File : ToFile  Filename=VRU_simout  MatrixName=VRU_simout  SampleTime=1/Mainfreq
  To File1 : ToFile  Filename=VRU_EGO_State_Flag06  MatrixName=VRU_EGO_State_Flag06  SampleTime=1/Mainfreq
  To File2 : ToFile  Filename=VRU_EGO_State_BrakeVel  MatrixName=VRU_EGO_State_BrakeVel  SampleTime=1/Mainfreq
  To Workspace : ToWorkspace  VariableName=VRU_EGO_State_Flag06  SampleTime=-1
      settings: MaxDataPoints=1
  To Workspace1 : ToWorkspace  VariableName=VRU_EGO_State_BrakeVel  SampleTime=1/Mainfreq
      settings: MaxDataPoints=1
  To Workspace2 : ToWorkspace  VariableName=VRU_simout  SaveFormat=Structure With Time  SampleTime=0.04
  wires:
  Mux/1 -> Data Type Conversion2/1
  Mux1/1 -> Data Type Conversion4/1
  Data Type Conversion4/1 -> Mux/3  "Flags"
  Ax/1 -> Rate Transition5/1
  Rate Transition5/1 -> Mux/2  "Ax"
  Switch1/1 -> Mux/4  "TTC"
  Constant/1 -> Switch1/1
  V/1 -> Mux/1  "V"
  det/1 -> Mux1/1
  warn/1 -> Mux1/2
  brake/1 -> Mux1/3, Data Type Conversion1/1, To Workspace/1  "VRU_EGO_State_Flag06"
  ped/1 -> Mux1/4
  ttc/1 -> Switch1/2, Switch1/3
  Coll/1 -> Data Type Conversion3/1, To Workspace1/1  "VRU_EGO_State_BrakeVel"
  Data Type Conversion1/1 -> To File1/1
  Data Type Conversion2/1 -> To File/1, To Workspace2/1
  Data Type Conversion3/1 -> To File2/1

== system PPS_Model/PPS Model/PPS_Radar/Radar ==
  Range : Inport
  Theta : Inport  Port=2
  All flags : Inport  Port=3
  Flag 0.6 : Inport  Port=4
  Enable : EnablePort
  DISPLAY1 : M-S-Function  FunctionName=msfcn_PPS_radar_graph  Parameters=RadarFreq TISdet RadarSwitch TISMaxRange TISMaxTheta*pi/180
  Degrees to Radians : simulink_extras/Transformations/Degrees to Radians
  wires:
  Range/1 -> DISPLAY1/1
  Theta/1 -> Degrees to Radians/1
  All flags/1 -> DISPLAY1/3
  Flag 0.6/1 -> DISPLAY1/4
  Degrees to Radians/1 -> DISPLAY1/2

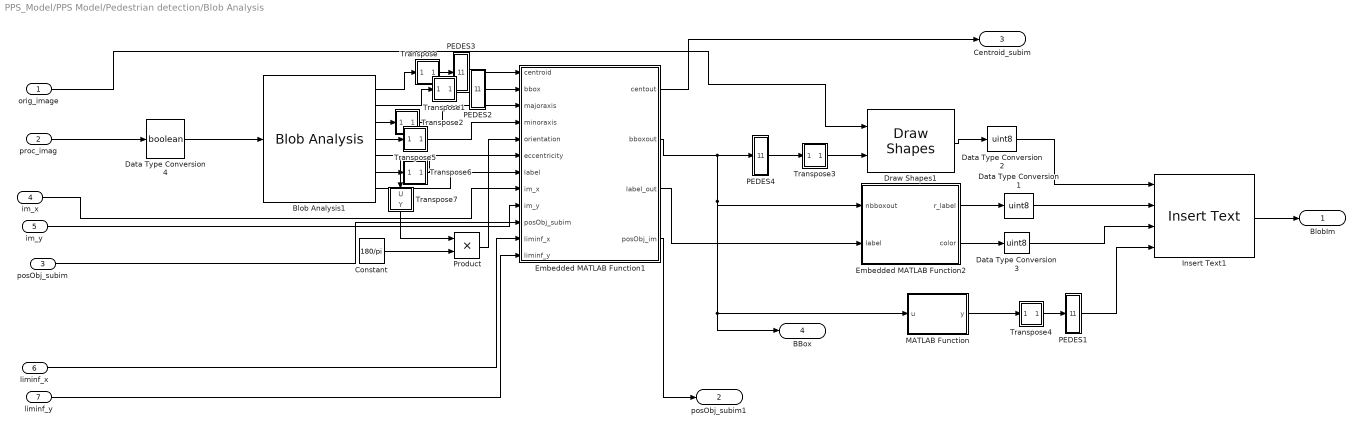
== system PPS_Model/PPS Model/Pedestrian detection/Blob Analysis ==
  orig_image : Inport
  proc_imag : Inport  Port=2
  posObj_subim : Inport  Port=3
  im_x : Inport  Port=4
  im_y : Inport  Port=5
  liminf_x : Inport  Port=6
  liminf_y : Inport  Port=7
  Blob Analysis1 : visionstatistics/Blob Analysis  Tag=vipblks_row_conv  area=off  centroid=on  bBox=on  majorAxis=on  minorAxis=on  angle=on  eccentricity=on  equivDiameterSq=off  extent=off  perimeter=off  maxBlobs=100  warnIfNumBlobsExceeded=on  isCount=off  useMinArea=on  minArea=50  useMaxArea=on  maxArea=150000  excludeBorderBlob=off  outDT=single  isOutVarDim=off  isFill=on  fillValues=-1  conn=4  isLabel=on  outputMode=Binary point scaling  outputWordLength=32  outputFracLength=16  firstCoeffMode=Binary point scaling  firstCoeffWordLength=16  firstCoeffFracLength=14  secondCoeffMode=Binary point scaling  secondCoeffWordLength=32  secondCoeffFracLength=16  accumMode=Binary point scaling  accumWordLength=32  accumFracLength=0  prodOutputMode=Binary point scaling  prodOutputWordLength=32  prodOutputFracLength=16  roundingMode=Floor  overflowMode=off
  Constant : Constant  Value=180/pi  VectorParams1D=off
  Data Type Conversion1 : DataTypeConversion  OutDataTypeStr=uint8
  Data Type Conversion2 : DataTypeConversion  OutDataTypeStr=uint8
  Data Type Conversion3 : DataTypeConversion  OutDataTypeStr=uint8
  Data Type Conversion4 : DataTypeConversion  OutDataTypeStr=boolean
  Draw Shapes1 : visiontextngfix/Draw Shapes  shape=Rectangles  fill=off  fillClrSource=Specify via dialog  display=White  intensity=200  color=[200 255 100]  opacity=0.6  viewport=Entire image  antialiasing=off  inType=Obsolete  imagePorts=One multidimensional signal  prodOutputMode=Binary point scaling  prodOutputWordLength=32  prodOutputFracLength=14  memoryMode=Specify word length  memoryWordLength=16  memoryFracLength=15  roundingMode=Floor  overflowMode=off
  Embedded MATLAB Function1 : MATLAB Function  TreatAsAtomicUnit=on
      settings: PermitHierarchicalResolution=ParametersOnly
  Embedded MATLAB Function2 : MATLAB Function  TreatAsAtomicUnit=on
      settings: PermitHierarchicalResolution=ParametersOnly
  Insert Text1 : visiontextngfix/Insert Text  inputType=Obsolete  theText='%02d'  getTextLocFrom=Input port  textLoc=[1 1]  getTextColorFrom=Input port  textColor=[0 0 0]  getTextIntensityFrom=Specify via dialog  textIntensity=0  getTextOpacityFrom=Specify via dialog  textOpacity=1.0  dummyVar2=0  dummyVar3=0  dummyVar4=0  imagePorts=One multidimensional signal  isInputTransposed=off  fontFace=LucidaSansRegular  dummyVar1=0  blockFontSize=12  antiAliased=on
  MATLAB Function : MATLAB Function  TreatAsAtomicUnit=on
      settings: PermitHierarchicalResolution=ParametersOnly
  PEDES1 : MATLAB Function  TreatAsAtomicUnit=on
      settings: PermitHierarchicalResolution=ParametersOnly
  PEDES2 : MATLAB Function  TreatAsAtomicUnit=on
      settings: PermitHierarchicalResolution=ParametersOnly
  PEDES3 : MATLAB Function  TreatAsAtomicUnit=on
      settings: PermitHierarchicalResolution=ParametersOnly
  PEDES4 : MATLAB Function  TreatAsAtomicUnit=on
      settings: PermitHierarchicalResolution=ParametersOnly
  Product : Product  RndMeth=Zero
  Transpose : Subsystem
  Transpose1 : Subsystem
  Transpose2 : Subsystem
  Transpose3 : Subsystem
  Transpose4 : Subsystem
  Transpose5 : Subsystem
  Transpose6 : Subsystem
  Transpose7 : Subsystem
  BlobIm : Outport
  posObj_subim1 : Outport  Port=2
  Centroid_subim : Outport  Port=3
  BBox : Outport  Port=4
  wires:
  Blob Analysis1/4 -> Transpose5/1(U)
  Constant/1 -> Product/2
  Embedded MATLAB Function2/1(r_label) -> Data Type Conversion1/1
  Embedded MATLAB Function2/2(color) -> Data Type Conversion3/1
  Draw Shapes1/1 -> Data Type Conversion2/1
  Data Type Conversion1/1 -> Insert Text1/2
  Data Type Conversion2/1 -> Insert Text1/1
  Data Type Conversion3/1 -> Insert Text1/3
  Blob Analysis1/1 -> Transpose/1(U)
  Blob Analysis1/2 -> Transpose1/1(U)
  Blob Analysis1/3 -> Transpose2/1(U)
  Blob Analysis1/5 -> Transpose7/1(U)
  Product/1 -> Embedded MATLAB Function1/5(orientation)
  Blob Analysis1/7 -> Embedded MATLAB Function1/7(label)
  Embedded MATLAB Function1/3(label_out) -> Embedded MATLAB Function2/2(label)
  Embedded MATLAB Function1/2(bboxout) -> Embedded MATLAB Function2/1(nbboxout), BBox/1, MATLAB Function/1(u), PEDES4/1(pts)
  Embedded MATLAB Function1/1(centout) -> Centroid_subim/1
  Insert Text1/1 -> BlobIm/1
  proc_imag/1 -> Data Type Conversion4/1
  im_x/1 -> Embedded MATLAB Function1/8(im_x)
  orig_image/1 -> Draw Shapes1/1
  im_y/1 -> Embedded MATLAB Function1/9(im_y)
  liminf_x/1 -> Embedded MATLAB Function1/11(liminf_x)
  liminf_y/1 -> Embedded MATLAB Function1/12(liminf_y)
  posObj_subim/1 -> Embedded MATLAB Function1/10(posObj_subim)
  Embedded MATLAB Function1/4(posObj_im) -> posObj_subim1/1
  Data Type Conversion4/1 -> Blob Analysis1/1
  Blob Analysis1/6 -> Transpose6/1(U)
  PEDES1/1(inpoints) -> Insert Text1/4
  Transpose/1(Y) -> PEDES3/1(pts)
  Transpose1/1(Y) -> PEDES2/1(pts)
  Transpose3/1(Y) -> Draw Shapes1/2
  PEDES2/1(inpoints) -> Embedded MATLAB Function1/2(bbox)
  PEDES3/1(inpoints) -> Embedded MATLAB Function1/1(centroid)
  Transpose4/1(Y) -> PEDES1/1(pts)
  PEDES4/1(inpoints) -> Transpose3/1(U)
  Transpose7/1(Y) -> Product/1
  Transpose6/1(Y) -> Embedded MATLAB Function1/6(eccentricity)
  Transpose5/1(Y) -> Embedded MATLAB Function1/4(minoraxis)
  Transpose2/1(Y) -> Embedded MATLAB Function1/3(majoraxis)
  MATLAB Function/1(y) -> Transpose4/1(U)

== system PPS_Model/PPS Model/Pedestrian detection/Image processing ==
  Image : Inport
  Closing : visionmorphops/Closing  nhoodsrc=Specify via dialog  strel=strel('disk', 4)
  Edge Detection : visionanalysis/Edge Detection  method=Canny  outputType=Binary image  userDefinedThreshold=off  thresholdSource=Specify via dialog  threshold=1  thresholdTuning=3  edgeThinning=off  threshold_canny=[0.25 0.60]  autoPercent=93  sigma=1  prodOutputMode=Binary point scaling  prodOutputWordLength=32  prodOutputFracLength=8  roundingMode=Floor  overflowMode=off
  Embedded MATLAB Function : MATLAB Function  TreatAsAtomicUnit=on
      settings: PermitHierarchicalResolution=ParametersOnly
  Image Data Type Conversion1 : visionconversions/Image Data Type Conversion  outDT=single  isSigned=on  wordLen=16  numFracBits=0
  ProcIm : Outport
  wires:
  Closing/1 -> Embedded MATLAB Function/1(image)
  Embedded MATLAB Function/1(im) -> ProcIm/1
  Image/1 -> Image Data Type Conversion1/1
  Edge Detection/1 -> Closing/1
  Image Data Type Conversion1/1 -> Edge Detection/1

== system PPS_Model/PPS Model/Pedestrian detection/Transpose1 ==
  U : Inport
  Data Type Conversion : DataTypeConversion
  Data Type Conversion1 : DataTypeConversion
  Interpreted MATLAB Function : MATLABFcn  MATLABFcn=transpose  Output1D=off
  Y : Outport
  wires:
  Data Type Conversion1/1 -> Y/1
  Interpreted MATLAB Function/1 -> Data Type Conversion1/1
  Data Type Conversion/1 -> Interpreted MATLAB Function/1
  U/1 -> Data Type Conversion/1

== system PPS_Model/PPS Model/Pedestrian detection/Transpose2 ==
  U : Inport
  Data Type Conversion : DataTypeConversion
  Data Type Conversion1 : DataTypeConversion
  Interpreted MATLAB Function : MATLABFcn  MATLABFcn=transpose  Output1D=off
  Y : Outport
  wires:
  U/1 -> Data Type Conversion/1
  Data Type Conversion/1 -> Interpreted MATLAB Function/1
  Interpreted MATLAB Function/1 -> Data Type Conversion1/1
  Data Type Conversion1/1 -> Y/1

== system PPS_Model/PPS Model/Pedestrian detection/Transpose3 ==
  U : Inport
  Data Type Conversion : DataTypeConversion
  Data Type Conversion1 : DataTypeConversion
  Interpreted MATLAB Function : MATLABFcn  MATLABFcn=transpose  Output1D=off
  Y : Outport
  wires:
  Data Type Conversion1/1 -> Y/1
  Interpreted MATLAB Function/1 -> Data Type Conversion1/1
  Data Type Conversion/1 -> Interpreted MATLAB Function/1
  U/1 -> Data Type Conversion/1

== system PPS_Model/PPS Model/Pedestrian detection/Transpose8 ==
  U : Inport
  Data Type Conversion : DataTypeConversion
  Data Type Conversion1 : DataTypeConversion
  Interpreted MATLAB Function : MATLABFcn  MATLABFcn=transpose  Output1D=off
  Y : Outport
  wires:
  Data Type Conversion1/1 -> Y/1
  Interpreted MATLAB Function/1 -> Data Type Conversion1/1
  Data Type Conversion/1 -> Interpreted MATLAB Function/1
  U/1 -> Data Type Conversion/1

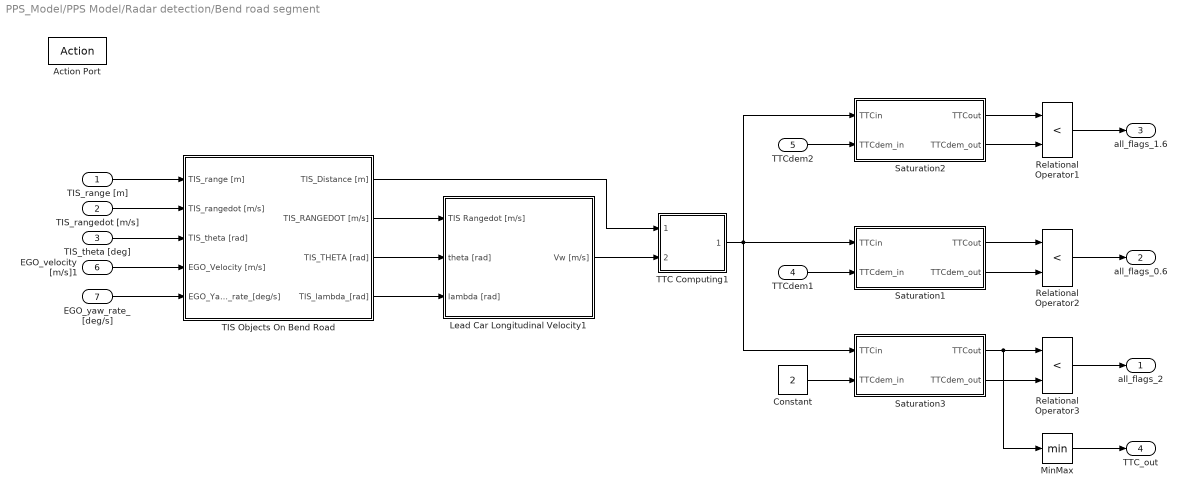
== system PPS_Model/PPS Model/Radar detection/Bend road segment ==
  TIS_range [m] : Inport  PortDimensions=TISdet
  TIS_rangedot [m/s] : Inport  Port=2  PortDimensions=TISdet
  TIS_theta [deg] : Inport  Port=3  PortDimensions=TISdet
  TTCdem1 : Inport  Port=4
  TTCdem2 : Inport  Port=5
  EGO_velocity [m/s]1 : Inport  Port=6
  EGO_yaw_rate_[deg/s] : Inport  Port=7
  Action Port : ActionPort  ActionType=then
  Constant : Constant  Value=2
  Lead Car Longitudinal Velocity1 : Subsystem
  MinMax : MinMax
  Relational Operator1 : RelationalOperator  Operator=<  OutDataTypeStr=fixdt(1,16)
  Relational Operator2 : RelationalOperator  Operator=<  OutDataTypeStr=fixdt(1,16)
  Relational Operator3 : RelationalOperator  Operator=<  OutDataTypeStr=fixdt(1,16)
  Saturation1 : Subsystem
  Saturation2 : Subsystem
  Saturation3 : Subsystem
  TIS Objects On Bend Road : Subsystem
  TTC Computing1 : Subsystem
  all_flags_2 : Outport  InitialOutput=0
  all_flags_0.6 : Outport  Port=2  InitialOutput=0
  all_flags_1.6 : Outport  Port=3  InitialOutput=zeros(TISdet,1)
  TTC_out : Outport  Port=4
  wires:
  EGO_yaw_rate_[deg/s]/1 -> TIS Objects On Bend Road/5(EGO_Yaw_rate_[deg/s])
  Lead Car Longitudinal Velocity1/1(Vw [m/s]) -> TTC Computing1/2(Velocity [m/s])
  EGO_velocity [m/s]1/1 -> TIS Objects On Bend Road/4(EGO_Velocity [m/s])
  TIS Objects On Bend Road/1(TIS_Distance [m]) -> TTC Computing1/1(Distance [m])
  TIS Objects On Bend Road/2(TIS_RANGEDOT [m/s]) -> Lead Car Longitudinal Velocity1/1(TIS Rangedot [m/s])
  TIS Objects On Bend Road/3(TIS_THETA [rad]) -> Lead Car Longitudinal Velocity1/2(theta [rad])
  TIS Objects On Bend Road/4(TIS_lambda_[rad]) -> Lead Car Longitudinal Velocity1/3(lambda [rad])
  TIS_range [m]/1 -> TIS Objects On Bend Road/1(TIS_range [m])
  TIS_rangedot [m/s]/1 -> TIS Objects On Bend Road/2(TIS_rangedot [m/s])
  TIS_theta [deg]/1 -> TIS Objects On Bend Road/3(TIS_theta [rad])
  TTC Computing1/1(TTC [s]) -> Saturation3/1(TTCin), Saturation1/1(TTCin), Saturation2/1(TTCin)
  Saturation2/1(TTCout) -> Relational Operator1/1
  Relational Operator1/1 -> all_flags_1.6/1
  TTCdem2/1 -> Saturation2/2(TTCdem_in)
  Saturation2/2(TTCdem_out) -> Relational Operator1/2
  Relational Operator2/1 -> all_flags_0.6/1
  TTCdem1/1 -> Saturation1/2(TTCdem_in)
  Saturation1/1(TTCout) -> Relational Operator2/1
  Saturation1/2(TTCdem_out) -> Relational Operator2/2
  MinMax/1 -> TTC_out/1
  Constant/1 -> Saturation3/2(TTCdem_in)
  Saturation3/2(TTCdem_out) -> Relational Operator3/2
  Saturation3/1(TTCout) -> Relational Operator3/1, MinMax/1
  Relational Operator3/1 -> all_flags_2/1

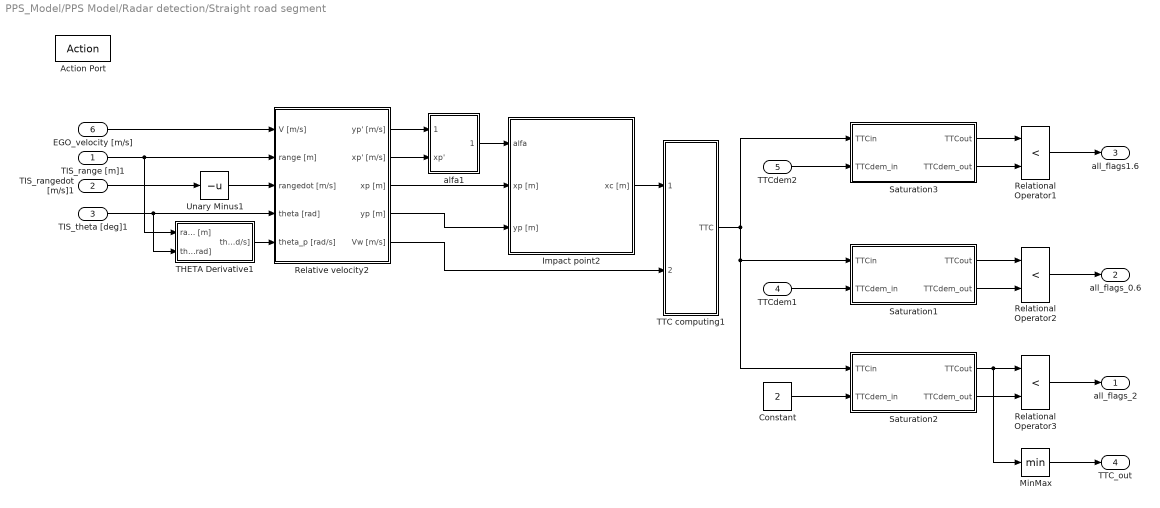
== system PPS_Model/PPS Model/Radar detection/Straight road segment ==
  TIS_range [m]1 : Inport  PortDimensions=TISdet
  TIS_rangedot [m/s]1 : Inport  Port=2  PortDimensions=TISdet
  TIS_theta [deg]1 : Inport  Port=3  PortDimensions=TISdet
  TTCdem1 : Inport  Port=4
  TTCdem2 : Inport  Port=5
  EGO_velocity [m/s] : Inport  Port=6
  Action Port : ActionPort  ActionType=else
  Constant : Constant  Value=2
  Impact point2 : Subsystem
  MinMax : MinMax
  Relational Operator1 : RelationalOperator  Operator=<  OutDataTypeStr=fixdt(1,16)
  Relational Operator2 : RelationalOperator  Operator=<  OutDataTypeStr=fixdt(1,16)
  Relational Operator3 : RelationalOperator  Operator=<  OutDataTypeStr=fixdt(1,16)
  Relative velocity2 : Subsystem
  Saturation1 : Subsystem
  Saturation2 : Subsystem
  Saturation3 : Subsystem
  THETA Derivative1 : Subsystem
  TTC computing1 : Subsystem
  Unary Minus1 : UnaryMinus
  alfa1 : Subsystem
  all_flags_2 : Outport  InitialOutput=0
  all_flags_0.6 : Outport  Port=2  SampleTime=1/TISfreq  InitialOutput=0
  all_flags1.6 : Outport  Port=3  SampleTime=1/TISfreq  InitialOutput=0
  TTC_out : Outport  Port=4
  wires:
  EGO_velocity [m/s]/1 -> Relative velocity2/1(V [m/s])
  TIS_range [m]1/1 -> THETA Derivative1/1(range [m]), Relative velocity2/2(range [m])
  TIS_rangedot [m/s]1/1 -> Unary Minus1/1
  TIS_theta [deg]1/1 -> Relative velocity2/4(theta [rad]), THETA Derivative1/2(theta [rad])
  THETA Derivative1/1(theta_dot [rad/s]) -> Relative velocity2/5(theta_p [rad/s])
  Relative velocity2/1(yp' [m/s]) -> alfa1/1(yp'1)
  Relative velocity2/2(xp' [m/s]) -> alfa1/2(xp')
  Relative velocity2/3(xp [m]) -> Impact point2/2(xp [m])
  alfa1/1(alfa1) -> Impact point2/1(alfa)
  Unary Minus1/1 -> Relative velocity2/3(rangedot [m/s])
  Relative velocity2/4(yp [m]) -> Impact point2/3(yp [m])
  Impact point2/1(xc [m]) -> TTC computing1/1(xc [m])
  Relative velocity2/5(Vw [m/s]) -> TTC computing1/2(Vw [m/s])
  TTC computing1/1(TTC) -> Saturation1/1(TTCin), Saturation2/1(TTCin), Saturation3/1(TTCin)
  Saturation3/1(TTCout) -> Relational Operator1/1
  Relational Operator1/1 -> all_flags1.6/1
  TTCdem2/1 -> Saturation3/2(TTCdem_in)
  Saturation3/2(TTCdem_out) -> Relational Operator1/2
  Relational Operator2/1 -> all_flags_0.6/1
  TTCdem1/1 -> Saturation1/2(TTCdem_in)
  Saturation1/1(TTCout) -> Relational Operator2/1
  Saturation1/2(TTCdem_out) -> Relational Operator2/2
  Constant/1 -> Saturation2/2(TTCdem_in)
  Saturation2/2(TTCdem_out) -> Relational Operator3/2
  Saturation2/1(TTCout) -> Relational Operator3/1, MinMax/1
  Relational Operator3/1 -> all_flags_2/1
  MinMax/1 -> TTC_out/1

== system PPS_Model/PPS Model/Radar detection/TIS1 Sorting  Fun ==
  TIS1range [m] : Inport
  TIS1rangedot [m/s] : Inport  Port=2
  TIS1theta [deg] : Inport  Port=3
  Degrees to Radians : simulink_extras/Transformations/Degrees to Radians
  Switch : Switch  Criteria=u2 ~= 0
  Unary Minus : UnaryMinus
  Unary Minus1 : UnaryMinus
  range max : Constant  Value=TISMaxRange
  TIS1_RANGE [m] : Outport
  TIS1_RANGEDOT [m/s] : Outport  Port=2
  TIS1_THETA [rad] : Outport  Port=3
  wires:
  Unary Minus/1 -> Degrees to Radians/1
  Switch/1 -> TIS1_RANGE [m]/1
  TIS1rangedot [m/s]/1 -> Unary Minus1/1
  range max/1 -> Switch/3
  Degrees to Radians/1 -> TIS1_THETA [rad]/1
  TIS1range [m]/1 -> Switch/1, Switch/2
  TIS1theta [deg]/1 -> Unary Minus/1
  Unary Minus1/1 -> TIS1_RANGEDOT [m/s]/1

== system PPS_Model/PPS Model/Pedestrian detection/Blob Analysis/Transpose ==
  U : Inport
  Data Type Conversion : DataTypeConversion
  Data Type Conversion1 : DataTypeConversion  OutDataTypeStr=single
  Interpreted MATLAB Function : MATLABFcn  MATLABFcn=transpose  Output1D=off
  Y : Outport
  wires:
  Data Type Conversion1/1 -> Y/1
  Interpreted MATLAB Function/1 -> Data Type Conversion1/1
  Data Type Conversion/1 -> Interpreted MATLAB Function/1
  U/1 -> Data Type Conversion/1
